simulink model "rot_pen_wok_sldrt"  (R2024a)
settings: Solver=ode1  StartTime=0.0  StopTime=inf  FixedStep=Ts  RelTol=1e-3
PostLoadFcn:
  | try
  | if isempty(which('ZHAWcbfcn'));
  | callback_fid07124=fopen('ZHAWcbfcn.m','w');
  | [~]=fprintf(callback_fid07124,'%s',get_param([bdroot,'/ Setup SLDRT'],'ClipboardFcn'));
  | [~]=fclose(callback_fid07124);
  | setpref('ZHAW_SLDRT_lib','cb_fcn',which('ZHAWcbfcn'))
  | clear callback_fid07124
  | end
  | catch
  | clear callback_fid07124
  | end
  | Ts=eval(get_param([bdroot,'/ Setup SLDRT'],'Ts'));
InitFcn:
  | Ts=eval(get_param([bdroot,'/ Setup SLDRT'],'Ts'));
values from neighbouring files (symbols this model uses):
  i_max = 1    [rot_pen_wok_ini.m]
  is_pendulum_up = 1    [rot_pen_wok_ini.m]
  Kp_i = db2mag(12)    [rot_pen_wok_ini.m]
  Kp_om = db2mag(-5) / 2    [rot_pen_wok_ini.m]
  Kp_phi2 = (k_sB2 + (k_sB1 - k_sB2) / 2) / 0.7961    [rot_pen_wok_ini.m]
  Kp_v = 0.0116    [rot_pen_wok_ini.m]
  om_max = 200    [rot_pen_wok_ini.m]
  phi2_disable = 10*pi/180    (= 0.174532925199)    [rot_pen_wok_ini.m]
  phi2_enable = 30*pi/180    (= 0.523598775598)    [rot_pen_wok_ini.m]
  phi2_max = 30 * pi/180    (= 0.523598775598)    [rot_pen_wok_ini.m]
  Tn_i = L/R    (= 0.00028905560459)    [rot_pen_wok_ini.m]
  Tn_om = 1/(2*pi*1)    (= 0.159154943092)    [rot_pen_wok_ini.m]
  Tn_phi2 = 1 / 18    (= 0.0555555555556)    [rot_pen_wok_ini.m]
  u_max = 24    [rot_pen_wok_ini.m]
undefined symbols (not defined in the file or in its folder): National_Instruments, PCIe, Tn_v
libraries: sldrtlib x5, cstblocks x2, simulink x1
(part 2 of 2)

== system rot_pen_wok_sldrt/ Setup SLDRT ==
  Real-Time Sync : Subsystem
  Synchronization : Constant
  wires:
  Synchronization/1 -> Real-Time Sync/Enable

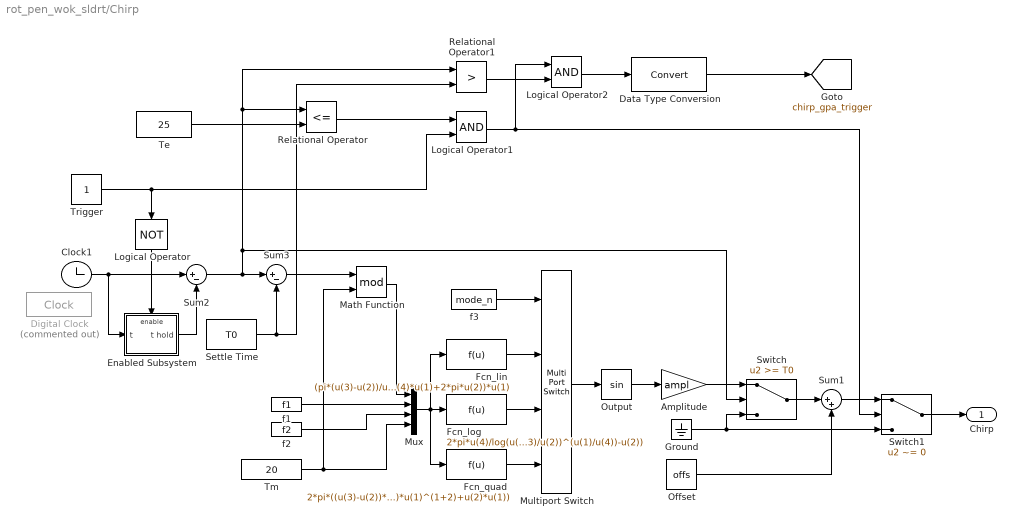
== system rot_pen_wok_sldrt/Chirp ==
  Amplitude : Gain  Gain=ampl
  Clock1 : Clock
      settings: DisableCoverage=on
  Data Type Conversion : DataTypeConversion  SaturateOnIntegerOverflow=off  RndMeth=Floor
  Digital Clock : DigitalClock  Commented=on  SampleTime=Ts
  Enabled Subsystem : Subsystem  TreatAsAtomicUnit=on
  Fcn_lin : Fcn  Expr=(pi*(u(3)-u(2))/u(4)*u(1)+2*pi*u(2))*u(1)
  Fcn_log : Fcn  Expr=2*pi*u(4)/log(u(3)/u(2))*(u(2)*(u(3)/u(2))^(u(1)/u(4))-u(2))
  Fcn_quad : Fcn  Expr=2*pi*((u(3)-u(2))*u(4)^(-2)/(1+2)*u(1)^(1+2)+u(2)*u(1))
  Ground : Ground
  Logical Operator : Logic  Operator=NOT  AllPortsSameDT=off  OutDataTypeStr=boolean
  Logical Operator1 : Logic  AllPortsSameDT=off
  Logical Operator2 : Logic  AllPortsSameDT=off
  Math Function : Math  Operator=mod  SignedPower=on
  Multiport Switch : MultiPortSwitch  SaturateOnIntegerOverflow=off  InputSameDT=off
  Mux : Mux
  Offset : Constant  Value=offs
  Output : Trigonometry
  Relational Operator : RelationalOperator  Operator=<=  RndMeth=Simplest  InputSameDT=off
  Relational Operator1 : RelationalOperator  Operator=>  RndMeth=Simplest  InputSameDT=off
  Settle Time : Constant  Value=T0
  Sum1 : Sum  Inputs=|++
  Sum2 : Sum  Inputs=|+-
  Sum3 : Sum  Inputs=|+-
  Switch : Switch  Threshold=T0  SaturateOnIntegerOverflow=off  InputSameDT=off
  Switch1 : Switch  Criteria=u2 ~= 0  SaturateOnIntegerOverflow=off  InputSameDT=off
  Te : Constant  Value=25
  Tm : Constant  Value=20
  Trigger : Constant
  f1 : Constant  Value=f1
  f2 : Constant  Value=f2
  f3 : Constant  Value=mode_n
  Chirp : Outport  VectorParamsAs1DForOutWhenUnconnected=off
  tag scope: chirp_gpa_trigger=global
  wires:
  Te/1 -> Relational Operator/2
  Logical Operator/1 -> Enabled Subsystem/Enable
  Enabled Subsystem/1(t hold) -> Sum2/2
  Trigger/1 -> Logical Operator1/2, Logical Operator/1
  f3/1 -> Multiport Switch/1
  Fcn_lin/1 -> Multiport Switch/2
  Fcn_log/1 -> Multiport Switch/3
  Fcn_quad/1 -> Multiport Switch/4
  Multiport Switch/1 -> Output/1
  Math Function/1 -> Mux/1
  f2/1 -> Mux/3
  f1/1 -> Mux/2
  Mux/1 -> Fcn_log/1, Fcn_lin/1, Fcn_quad/1
  Clock1/1 -> Enabled Subsystem/1(t), Sum2/1
  Output/1 -> Amplitude/1
  Offset/1 -> Sum1/2
  Sum3/1 -> Math Function/1
  Tm/1 -> Mux/4, Math Function/2
  Switch/1 -> Sum1/1
  Amplitude/1 -> Switch/1
  Ground/1 -> Switch1/3, Switch/3
  Settle Time/1 -> Relational Operator1/2, Sum3/2
  Sum2/1 -> Switch/2, Relational Operator1/1, Relational Operator/1, Sum3/1
  Switch1/1 -> Chirp/1
  Sum1/1 -> Switch1/1
  Relational Operator/1 -> Logical Operator1/1
  Logical Operator1/1 -> Logical Operator2/1, Switch1/2
  Logical Operator2/1 -> Data Type Conversion/1
  Data Type Conversion/1 -> [chirp_gpa_trigger]
  Relational Operator1/1 -> Logical Operator2/2

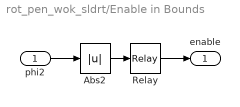
== system rot_pen_wok_sldrt/Enable in Bounds ==
  phi2 : Inport
  Abs2 : Abs  SaturateOnIntegerOverflow=off
  Relay : Relay  OnSwitchValue=phi2_enable  OffSwitchValue=phi2_disable  OnOutputValue=0  OffOutputValue=1
  enable : Outport
  wires:
  Abs2/1 -> Relay/1
  phi2/1 -> Abs2/1
  Relay/1 -> enable/1

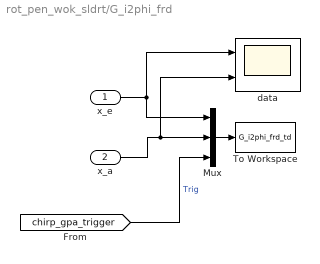
== system rot_pen_wok_sldrt/G_i2phi_frd ==
  x_e : Inport
  x_a : Inport  Port=2
  Mux : Mux  Inputs=3
  To Workspace : ToWorkspace  VariableName=G_i2phi_frd_td  SaveFormat=Structure With Time  SampleTime=Ts
  data : Scope  NumInputPorts=2
      settings: CopyFcn=try ZHAWcbfcn('copyScope'); end  NameChangeFcn=try ZHAWcbfcn('namechangeScope'); end
  wires:
  x_e/1 -> data/1, Mux/1
  x_a/1 -> data/2, Mux/2
  Mux/1 -> To Workspace/1
  [chirp_gpa_trigger] -> Mux/3  "Trig"

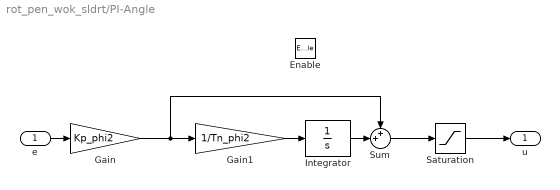
== system rot_pen_wok_sldrt/PI-Angle ==
  e : Inport
  Enable : EnablePort  StatesWhenEnabling=reset
  Gain : Gain  Gain=Kp_phi2
  Gain1 : Gain  Gain=1/Tn_phi2
  Integrator : Integrator  LimitOutput=on  UpperSaturationLimit=om_max  LowerSaturationLimit=-om_max
  Saturation : Saturate  UpperLimit=om_max  LowerLimit=-om_max
  Sum : Sum  Inputs=++|
  u : Outport  OutputWhenDisabled=reset  InitialOutput=0
  wires:
  Gain/1 -> Gain1/1, Sum/1
  Saturation/1 -> u/1
  Sum/1 -> Saturation/1
  Integrator/1 -> Sum/2
  Gain1/1 -> Integrator/1
  e/1 -> Gain/1

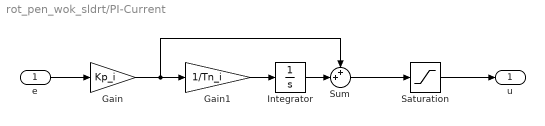
== system rot_pen_wok_sldrt/PI-Current ==
  e : Inport
  Gain : Gain  Gain=Kp_i
  Gain1 : Gain  Gain=1/Tn_i
  Integrator : Integrator  LimitOutput=on  UpperSaturationLimit=u_max  LowerSaturationLimit=-u_max
  Saturation : Saturate  UpperLimit=u_max  LowerLimit=-u_max
  Sum : Sum  Inputs=++|
  u : Outport
  wires:
  Gain1/1 -> Integrator/1
  e/1 -> Gain/1
  Integrator/1 -> Sum/2
  Gain/1 -> Gain1/1, Sum/1
  Sum/1 -> Saturation/1
  Saturation/1 -> u/1

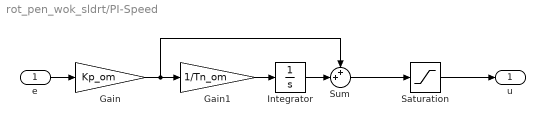
== system rot_pen_wok_sldrt/PI-Speed ==
  e : Inport
  Gain : Gain  Gain=Kp_om
  Gain1 : Gain  Gain=1/Tn_om
  Integrator : Integrator  LimitOutput=on  UpperSaturationLimit=i_max  LowerSaturationLimit=-i_max
  Saturation : Saturate  UpperLimit=i_max  LowerLimit=-i_max
  Sum : Sum  Inputs=++|
  u : Outport
  wires:
  Saturation/1 -> u/1
  Sum/1 -> Saturation/1
  Gain/1 -> Gain1/1, Sum/1
  Integrator/1 -> Sum/2
  e/1 -> Gain/1
  Gain1/1 -> Integrator/1

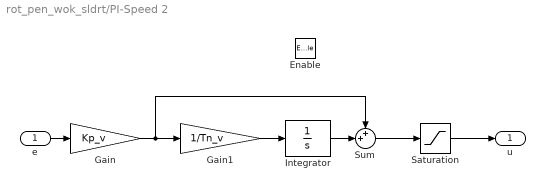
== system rot_pen_wok_sldrt/PI-Speed 2 ==
  e : Inport
  Enable : EnablePort  StatesWhenEnabling=reset
  Gain : Gain  Gain=Kp_v
  Gain1 : Gain  Gain=1/Tn_v
  Integrator : Integrator  LimitOutput=on  UpperSaturationLimit=phi2_max  LowerSaturationLimit=-phi2_max
  Saturation : Saturate  UpperLimit=phi2_max  LowerLimit=-phi2_max
  Sum : Sum  Inputs=++|
  u : Outport  OutputWhenDisabled=reset  InitialOutput=0
  wires:
  e/1 -> Gain/1
  Gain1/1 -> Integrator/1
  Integrator/1 -> Sum/2
  Sum/1 -> Saturation/1
  Saturation/1 -> u/1
  Gain/1 -> Sum/1, Gain1/1

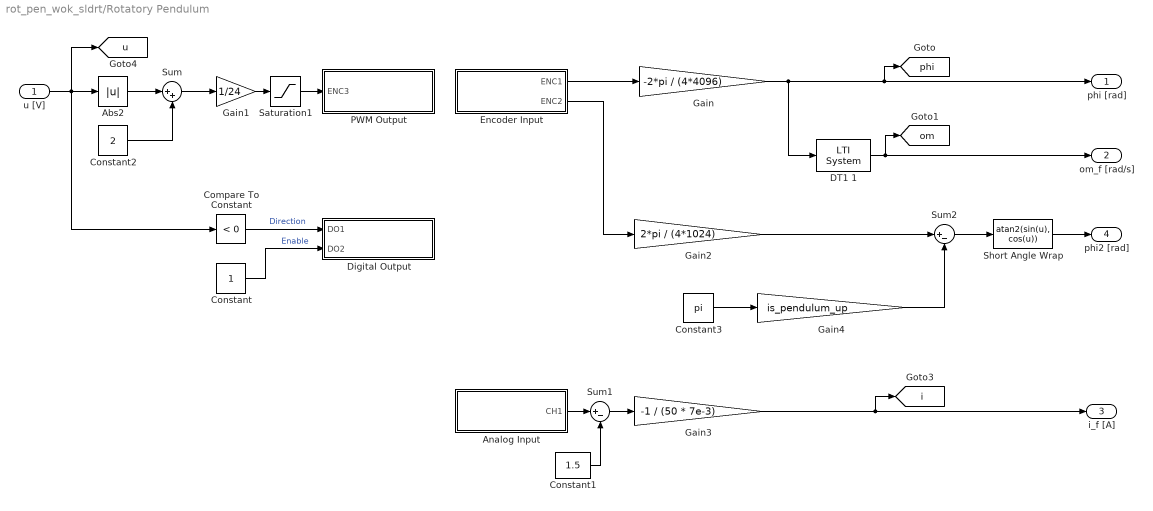
== system rot_pen_wok_sldrt/Rotatory Pendulum ==
  u [V] : Inport
  Abs2 : Abs  SaturateOnIntegerOverflow=off
  Analog Input : Subsystem  mask(NI Analog Input){device=PCIe-6321, connect=Banana Terminal, couple=differential, ch1=on, ch9=off, ch2=off, ch10=off, ch3=off, ch11=off, ch4=off, ch12=off, ch5=off, ch13=off, ch6=off, ch14=off, ch7=off, ch15=off, ch8=off, ch16=off, Ts=Ts}
      mask prompts: device "NI Device Type:"; connect "Connector Box:"; couple "CH Coupling:"; ch1 "CH1-CH9"; ch9 "CH9-GND"; ch2 "CH2-CH10"; ch10 "CH10-GND"; ch3 "CH3-CH11"; ch11 "CH11-GND"; ch4 "CH4-CH12"; ch12 "CH12-GND"; ch5 "CH5-CH13"; ch13 "CH13-GND"; ch6 "CH6-CH14"; ch14 "CH14-GND"; ch7 "CH7-CH15"; ch15 "CH15-GND"; ch8 "CH8-CH16"; ch16 "CH16-GND"; Ts "Sample Time:"
      mask help:
      | AD Converter
      | +/-10V
      mask init:
      | try ch_list = ZHAWcbfcn('get_ch_list'); end
      | try ZHAWcbfcn('BlockUpdate'); end
      settings: AttributesFormatString=%<couple>  OpenFcn=try ZHAWcbfcn('openMask'); end
      settings: CopyFcn=|
      | try
      | ZHAWcbfcn('CopyIOblock')
      | end
      | set_param(gcb,'OpenFcn','try ZHAWcbfcn(''openMask''); end')
      mask TypeOptions device: PCI-6221 | PCI-6259 | PCIe-6259 | PCIe-6321 | PCIe-6363
      mask TypeOptions connect: BNC Terminal | Banana Terminal | Screw Terminal
      mask Callback connect:
      | try ZHAWcbfcn('SetConnectorBox'); end
      | try ZHAWcbfcn('SetChannelCoupling'); end
      mask TypeOptions couple: single ended | differential
      mask Callback couple:
      | try ZHAWcbfcn('SetChannelCoupling'); end
      | try ZHAWcbfcn('SetConnectorBox'); end
      mask DialogControl DescGroupVar Prompt: NI Analog Input (R2024a)
      mask Display: disp('NI\nPCIe-6321')
  Compare To Constant : simulink/Logic and Bit Operations/Compare To Constant  relop=<  const=0  OutDataTypeStr=boolean
  Constant : Constant
  Constant1 : Constant  Value=1.5
  Constant2 : Constant  Value=2
  Constant3 : Constant  Value=pi
  DT1 1 : cstblocks/LTI System  sys=G_phi2omf  IC=[]  PadeOrder=0
  Digital Output : Subsystem  mask(NI Digital Output){device=PCIe-6321, connect=Banana Terminal, ch1=on, ch2=on, ch3=off, ch4=off, ch5=off, ch6=off, ch7=off, ch8=off, Ts=Ts}
      mask prompts: device "NI Device Type:"; connect "Connector Box:"; ch1 "DO1"; ch2 "DO2"; ch3 "DO3"; ch4 "DO4"; ch5 "DO5"; ch6 "DO6"; ch7 "DO7"; ch8 "DO8"; Ts "Sample Time:"
      mask help: Digital output 5V TTL.
      mask init:
      | try ch_list = ZHAWcbfcn('get_ch_list'); end
      | try ZHAWcbfcn('BlockUpdate'); end
      settings: OpenFcn=try ZHAWcbfcn('openMask'); end
      settings: CopyFcn=|
      | try
      | ZHAWcbfcn('CopyIOblock')
      | end
      | set_param(gcb,'OpenFcn','try ZHAWcbfcn(''openMask''); end')
      mask TypeOptions device: PCI-6221 | PCI-6259 | PCIe-6259 | PCIe-6321 | PCIe-6363
      mask Callback device: try ZHAWcbfcn('SetChannelNumber'); end
      mask TypeOptions connect: BNC Terminal | Banana Terminal | Screw Terminal
      mask Callback connect: try ZHAWcbfcn('SetConnectorBox'); end
      mask DialogControl DescGroupVar Prompt: NI Digital Output (R2024a)
      mask Display: disp('NI\nPCIe-6321')
  Encoder Input : Subsystem  mask(NI Encoder Input){device=PCIe-6321, connect=Banana Terminal, reset=off, ch1=on, ch2=on, ch3=off, ch4=off, Ts=Ts}
      mask prompts: device "NI Device Type:"; connect "Connector Box:"; reset "Reset at Index:"; ch1 "ENC1"; ch2 "ENC2"; ch3 "ENC3"; ch4 "ENC4"; Ts "Sample Time:"
      mask help:
      | Quadratur Encoder.
      | X4 Decoding.
      | Output is increments.
      mask init:
      | try ch_list = ZHAWcbfcn('get_ch_list'); end
      | try ZHAWcbfcn('BlockUpdate'); end
      settings: AttributesFormatString=Index Reset: %<reset>  OpenFcn=try ZHAWcbfcn('openMask'); end
      settings: CopyFcn=|
      | try
      | ZHAWcbfcn('CopyIOblock')
      | end
      | set_param(gcb,'OpenFcn','try ZHAWcbfcn(''openMask''); end')
      mask TypeOptions device: PCI-6221 | PCI-6259 | PCIe-6259 | PCIe-6321 | PCIe-6363
      mask Callback device: try ZHAWcbfcn('SetChannelNumber'); end
      mask TypeOptions connect: BNC Terminal | Banana Terminal | Screw Terminal
      mask Callback connect: try ZHAWcbfcn('SetConnectorBox'); end
      mask TypeOptions reset: on | off
      mask Callback reset: try ZHAWcbfcn('SetEncoderReset'); end
      mask DialogControl DescGroupVar Prompt: NI Encoder Input (R2024a)
      mask Display: disp('NI\nPCIe-6321')
  Gain : Gain  Gain=-2*pi / (4*4096)
  Gain1 : Gain  Gain=1/24
  Gain2 : Gain  Gain=2*pi / (4*1024)
  Gain3 : Gain  Gain=-1 / (50 * 7e-3)
  Gain4 : Gain  Gain=is_pendulum_up
  PWM Output : Subsystem  mask(NI PWM Output){device=PCIe-6321, connect=Banana Terminal, mode=PWM, ch1=off, ch2=off, ch3=on, ch4=off, pwm_frequ=20e3, duty=0, Ts_copy=Ts}
      mask prompts: device "NI Device Type:"; connect "Connector Box :"; mode "Output Modus:"; ch1 "ENC1"; ch2 "ENC2"; ch3 "ENC3"; ch4 "ENC4"; pwm_frequ "PWM Frequency [Hz]:"; duty "Duty Cycle [0...1]:"; Ts_copy "Sample Time:"
      mask help:
      | PWM or Frequency output.
      |
      | PWM:
      | The input specifies the duty cycle as a decimal fraction from 0 through 1 inclusive.
      | It determines the amount of time that the output signal value is high (1).
      |
      | Frequency;
      | The input specifies the output frequency in [Hz].
      mask init:
      | try ch_list = ZHAWcbfcn('get_ch_list'); end
      | try ZHAWcbfcn('BlockUpdate'); end
      settings: OpenFcn=try ZHAWcbfcn('openMask'); end
      settings: CopyFcn=|
      | try
      | ZHAWcbfcn('CopyIOblock')
      | end
      | set_param(gcb,'OpenFcn','try ZHAWcbfcn(''openMask''); end')
      mask TypeOptions device: PCI-6221 | PCI-6259 | PCIe-6259 | PCIe-6321 | PCIe-6363
      mask Callback device: try ZHAWcbfcn('SetChannelNumber'); end
      mask TypeOptions connect: BNC Terminal | Banana Terminal | Screw Terminal
      mask Callback connect: try ZHAWcbfcn('SetConnectorBox'); end
      mask TypeOptions mode: PWM | Frequency
      mask DialogControl DescGroupVar Prompt: NI Analog Output (R2024a)
      mask Display: disp('NI\nPCIe-6321')
  Saturation1 : Saturate  UpperLimit=1  LowerLimit=0
  Short Angle Wrap : Fcn  Expr=atan2(sin(u), cos(u))
  Sum : Sum  Inputs=|++
  Sum1 : Sum  Inputs=|+-
  Sum2 : Sum  Inputs=|+-
  phi [rad] : Outport
  om_f [rad/s] : Outport  Port=2
  i_f [A] : Outport  Port=3
  phi2 [rad] : Outport  Port=4
  tag scope: i=global, om=global, phi=global, u=global
  wires:
  Compare To Constant/1 -> Digital Output/1(DO1)  "Direction"
  Gain/1 -> [phi], phi [rad]/1, DT1 1/1
  Encoder Input/1(ENC1) -> Gain/1
  u [V]/1 -> Compare To Constant/1, Abs2/1, [u]
  Constant/1 -> Digital Output/2(DO2)  "Enable"
  Analog Input/1(CH1) -> Sum1/1
  Constant1/1 -> Sum1/2
  Sum1/1 -> Gain3/1
  Gain3/1 -> [i], i_f [A]/1
  DT1 1/1 -> [om], om_f [rad/s]/1
  Saturation1/1 -> PWM Output/1(ENC3)
  Abs2/1 -> Sum/1
  Sum/1 -> Gain1/1
  Constant2/1 -> Sum/2
  Gain1/1 -> Saturation1/1
  Encoder Input/2(ENC2) -> Gain2/1
  Gain2/1 -> Sum2/1
  Sum2/1 -> Short Angle Wrap/1
  Short Angle Wrap/1 -> phi2 [rad]/1
  Constant3/1 -> Gain4/1
  Gain4/1 -> Sum2/2

== system rot_pen_wok_sldrt/ Setup SLDRT/Real-Time Sync ==
  Enable : EnablePort
  Real-Time Synchronization : sldrtlib/Real-Time Synchronization  SampleTime=Ts  MaxMissedTicks=inf  ShowMissedTicks=off  YieldWhenWaiting=off

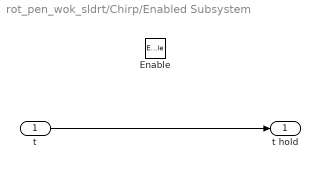
== system rot_pen_wok_sldrt/Chirp/Enabled Subsystem ==
  t : Inport
  Enable : EnablePort
  t hold : Outport  VectorParamsAs1DForOutWhenUnconnected=off
  wires:
  t/1 -> t hold/1

== system rot_pen_wok_sldrt/Rotatory Pendulum/Analog Input ==
  Analog Input : sldrtlib/Analog Input  SampleTime=Ts  MaxMissedTicks=10  ShowMissedTicks=off  YieldWhenWaiting=off  DrvName=National_Instruments/PCIe-6321  DrvAddress=4294967295  DrvOptions="[1  3  0  2  2  3  2]"  Channels=ch_list  RangeMode=1  VoltRange=1  DataType=1
      settings: AttributesFormatString=National Instruments\nPCIe-6321 [auto]
  Mux : Demux  Outputs=1
  CH1 : Outport  VectorParamsAs1DForOutWhenUnconnected=off
  wires:
  Mux/1 -> CH1/1
  Analog Input/1 -> Mux/1

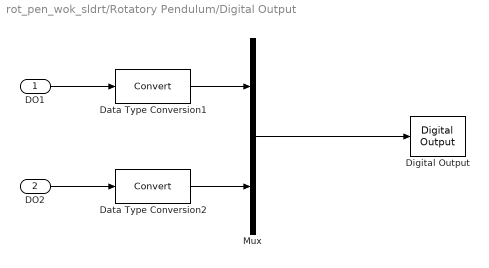
== system rot_pen_wok_sldrt/Rotatory Pendulum/Digital Output ==
  DO1 : Inport
  DO2 : Inport  Port=2
  Data Type Conversion1 : DataTypeConversion  SaturateOnIntegerOverflow=off  RndMeth=Floor
  Data Type Conversion2 : DataTypeConversion  SaturateOnIntegerOverflow=off  RndMeth=Floor
  Digital Output : sldrtlib/Digital Output  SampleTime=Ts  MaxMissedTicks=10  ShowMissedTicks=off  YieldWhenWaiting=off  DrvName=National_Instruments/PCIe-6321  DrvAddress=4294967295  DrvOptions="[1  3  0  2  2  3  2]"  Channels=ch_list  BitMode=1  InitialValue=0  FinalValue=0
      settings: AttributesFormatString=National Instruments\nPCIe-6321 [auto]
  Mux : Mux  Inputs=2
  wires:
  DO1/1 -> Data Type Conversion1/1
  DO2/1 -> Data Type Conversion2/1
  Mux/1 -> Digital Output/1
  Data Type Conversion1/1 -> Mux/1
  Data Type Conversion2/1 -> Mux/2

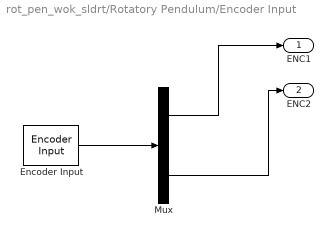
== system rot_pen_wok_sldrt/Rotatory Pendulum/Encoder Input ==
  Encoder Input : sldrtlib/Encoder Input  SampleTime=Ts  MaxMissedTicks=10  ShowMissedTicks=off  YieldWhenWaiting=off  DrvName=National_Instruments/PCIe-6321  DrvAddress=4294967295  DrvOptions="[1  3  0  2  2  3  2]"  Channels=ch_list  QuadMode=3  IndexPulse=1  InputFilter=Inf  DataType=1
      settings: AttributesFormatString=National Instruments\nPCIe-6321 [auto]
  Mux : Demux  Outputs=2
  ENC1 : Outport  VectorParamsAs1DForOutWhenUnconnected=off
  ENC2 : Outport  Port=2
  wires:
  Encoder Input/1 -> Mux/1
  Mux/1 -> ENC1/1
  Mux/2 -> ENC2/1

== system rot_pen_wok_sldrt/Rotatory Pendulum/PWM Output ==
  ENC3 : Inport
  Frequency Output : sldrtlib/Frequency Output  SampleTime=Ts  MaxMissedTicks=10  ShowMissedTicks=off  YieldWhenWaiting=off  DrvName=National_Instruments/PCIe-6321  DrvAddress=4294967295  DrvOptions="[1  3  0  2  2  3  2]"  Channels=ch_list  FrequencySource=1  Frequency=20e3  FrequencyFinalValue=20e3  DutySource=2  Duty=0  DutyFinalValue=0
      settings: AttributesFormatString=National Instruments\nPCIe-6321 [auto]
  Mux : Mux  Inputs=1
  wires:
  Mux/1 -> Frequency Output/1
  ENC3/1 -> Mux/1
